simulink model "ME322_Exercise_1_Simulink"  (R2024b)
settings: Solver=VariableStepAuto  StartTime=0.0  StopTime=10.0  RelTol=1e-3
undefined symbols (not defined in the file): A, b, k, M, m, phi, w
settings Model: Creator=clbonney  LastModifiedBy=Caide

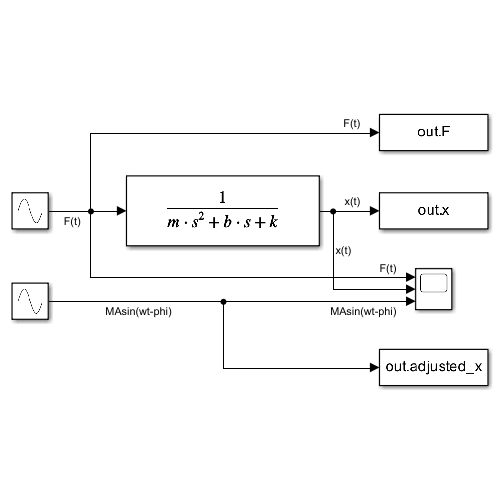
[thumbnail: Simulink's stored preview of the top-level diagram]
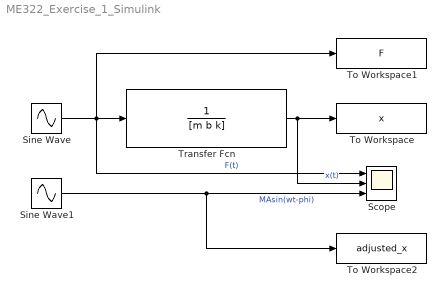
== system ME322_Exercise_1_Simulink ==
  Scope : Scope  NumInputPorts=3
  Sine Wave : Sin  Amplitude=A  Frequency=w  SampleTime=0
  Sine Wave1 : Sin  Amplitude=M*A  Frequency=w  Phase=phi  SampleTime=0
  To Workspace : ToWorkspace  VariableName=x  SampleTime=-1
  To Workspace1 : ToWorkspace  VariableName=F  SampleTime=-1
  To Workspace2 : ToWorkspace  VariableName=adjusted_x  SampleTime=-1
  Transfer Fcn : TransferFcn  Denominator=[m b k]
  wires:
  Transfer Fcn/1 -> Scope/2, To Workspace/1  "x(t)"
  Sine Wave/1 -> Scope/1, To Workspace1/1, Transfer Fcn/1  "F(t)"
  Sine Wave1/1 -> Scope/3, To Workspace2/1  "MAsin(wt-phi)"
